simulink model "Tutorial_Simulink_2"  (R2024a)
settings: Solver=FixedStepAuto  StartTime=0.0  StopTime=40  FixedStep=.1  RelTol=1e-3
settings Model: Creator=gzipprich  LastModifiedBy=gzipprich

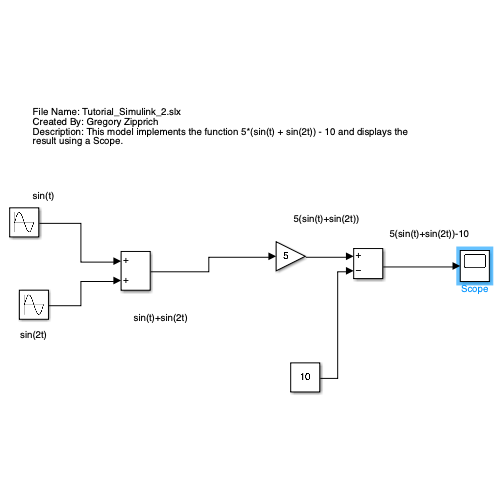
[thumbnail: Simulink's stored preview of the top-level diagram]
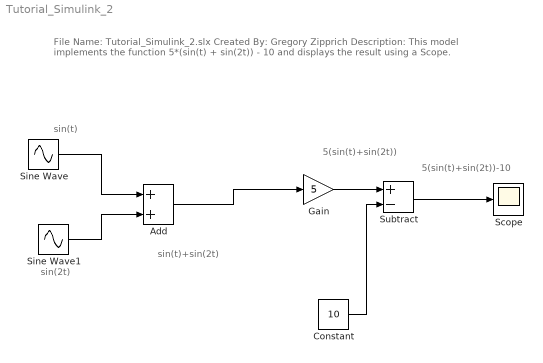
== system Tutorial_Simulink_2 ==
  note: File Name: Tutorial_Simulink_2.slx
      | Created By: Gregory Zipprich
      | Description: This model implements the function 5*(sin(t) + sin(2t)) - 10 and displays the result using a Scope.
  note: 5(sin(t)+sin(2t))-10
  note: 5(sin(t)+sin(2t))
  note: sin(t)+sin(2t)
  note: sin(2t)
  note: sin(t)
  Add : Sum
  Constant : Constant  Value=10
  Gain : Gain  Gain=5  ParamMin=[1]  ParamMax=[5]
  Scope : Scope
  Sine Wave : Sin  SampleTime=0
  Sine Wave1 : Sin  Frequency=2  SampleTime=0
  Subtract : Sum  Inputs=+-
  wires:
  Sine Wave/1 -> Add/1
  Sine Wave1/1 -> Add/2
  Add/1 -> Gain/1
  Constant/1 -> Subtract/2
  Gain/1 -> Subtract/1
  Subtract/1 -> Scope/1
